simulink model "rocky_model"  (R2020b)
settings: Solver=VariableStepAuto  StartTime=0.0  StopTime=15  RelTol=1e-3
values from neighbouring files (symbols this model uses):
  a = 12.5    [Rocky_closed_loop_poles.m]    (also in load_values.m; rocky_calibration.m = 1/(right_time_constant))
  b = 0.00323    [Rocky_closed_loop_poles.m]    (also in load_values.m; rocky_calibration.m = right_K)
  Ci = double(solutions.Ci)    [Rocky_closed_loop_poles.m]    (also in load_values.m = 659)
  g = 9.81    [Rocky_closed_loop_poles.m]    (also in cartpend_state_space.m = -10; load_values.m = 9.8; rocky_calibration.m = 9.8)
  JiCp = 598    [load_values.m]
  Jp = double(solutions.Jp)    [Rocky_closed_loop_poles.m]    (also in load_values.m = -12.38)
  Ki = double(solutions.Ki)    [Rocky_closed_loop_poles.m]    (also in load_values.m = 19.804)
  Kp = double(solutions.Kp)    [Rocky_closed_loop_poles.m]    (also in load_values.m = 4.086)
  l = 22*2.54/100    (= 0.5588)    [Rocky_closed_loop_poles.m]    (also in load_values.m = 0.4195)
undefined symbols (not defined in the file or in its folder): sigbuilder_block
settings Model: Creator=wsh32  LastModifiedBy=wsh32

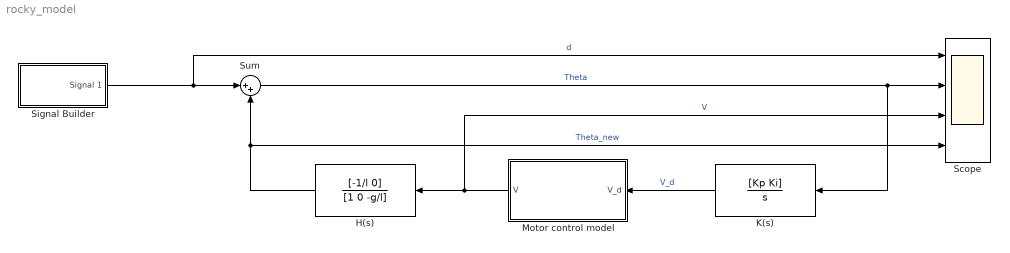
== system rocky_model ==
  H(s) : TransferFcn  Numerator=[-1/l 0]  Denominator=[1 0 -g/l]
  K(s) : TransferFcn  Numerator=[Kp Ki]  Denominator=[1 0]
  Motor control model : Subsystem
  Scope : Scope  NumInputPorts=4
  Signal Builder : Subsystem  Tag=STV Subsys  LoadFcn=sigbuilder_block('load');  StartFcn=sigbuilder_block('start');  StopFcn=sigbuilder_block('stop');  ClipboardFcn=sigbuilder_block('clipboard');  mask(Sigbuilder block){tuvar=[0:10]}
      mask help: Simulink:masks:SigbuilderBlock_MD
      mask init:
      | if ~strcmp(get_param(bdroot(gcbh),'SimulationStatus'),'stopped') tuvar = sigbuilder_block('maskInit'); end
      settings: CopyFcn=sigbuilder_block('copy');  DeleteFcn=sigbuilder_block('delete');  ModelCloseFcn=sigbuilder_block('modelClose');  PreSaveFcn=sigbuilder_block('preSave');  PauseFcn=sigbuilder_block('pause');  ContinueFcn=sigbuilder_block('continue');  NameChangeFcn=sigbuilder_block('namechange');  OpenFcn=sigbuilder_block('open',[437.6 199.2 550.4 400 ]);  CloseFcn=sigbuilder_block('close');
      mask Display: plot(0, 0, 100, 100,[2, 2, 32, 32, 2], [68, 8, 8, 68, 68],[32, 2], [38, 38], [32, 19, 2],[53, 60, 44], [32, 17, 17, 2],[16, 16, 31, 31]);txt = getActiveGroup(gcbh);text(2, 100, txt,'verticalAlignment', 'top');
  Sum : Sum  Inputs=|++
  wires:
  Signal Builder/1(Signal 1) -> Scope/1, Sum/1  "d"
  Sum/1 -> K(s)/1, Scope/2  "Theta"
  K(s)/1 -> Motor control model/1(V_d)  "V_d"
  H(s)/1 -> Sum/2, Scope/4  "Theta_new"
  Motor control model/1(V) -> H(s)/1, Scope/3  "V"

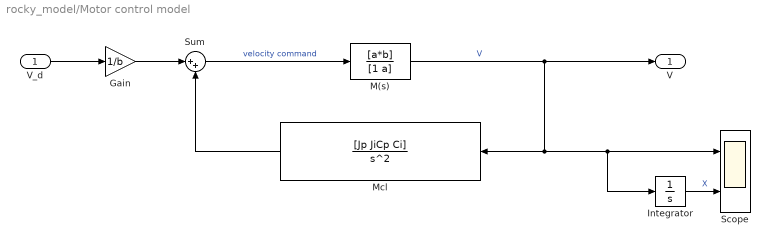
== system rocky_model/Motor control model ==
  V_d : Inport
  Gain : Gain  Gain=1/b
  Integrator : Integrator
  M(s) : TransferFcn  Numerator=[a*b]  Denominator=[1 a]
  Mcl : TransferFcn  Numerator=[Jp JiCp Ci]  Denominator=[1 0 0]
  Scope : Scope  NumInputPorts=2
  Sum : Sum  Inputs=|++
  V : Outport
  wires:
  Sum/1 -> M(s)/1  "velocity command"
  V_d/1 -> Gain/1
  M(s)/1 -> V/1, Integrator/1, Scope/1, Mcl/1  "V"
  Mcl/1 -> Sum/2
  Integrator/1 -> Scope/2  "X"
  Gain/1 -> Sum/1

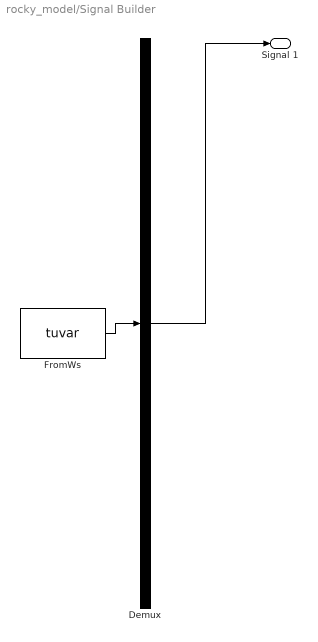
== system rocky_model/Signal Builder ==
  Demux : Demux  Tag=STV Demux  Outputs=1
      settings: DisplayOption=none
  FromWs : FromWorkspace  Tag=STV FromWs  VariableName=tuvar
      SigBuilderData=|
      | common.afterFinalStr = 'Extrapolate'
      | common.sampleTime = 0
      | dataSet.timeRange = [0 10]
      | dataSet.name = 'Group 1'
      | sbobj.Groups.Name = 'Group 1'
      | sbobj.Groups.Signals.Name = 'Signal 1'
      | sbobj.Groups.Signals.XData = [0 1 1 1.1 1.1 10]
      | sbobj.Groups.Signals.YData = [0 0 0.174532925199 0.174532925199 0 0]
  Signal 1 : Outport  Tag=STV Outport
  wires:
  Demux/1 -> Signal 1/1
  FromWs/1 -> Demux/1
